simulink model "PID"  (R2023b)
settings: Solver=VariableStepAuto  StartTime=0.0  StopTime=30  RelTol=1e-3
values from neighbouring files (symbols this model uses):
  A = double(A)    [consistent.m]    (also in dyn_model_mark.m)
  B = double(B)    [consistent.m]    (also in dyn_model_mark.m)
  C = [1 0 0 0 ... (first row only)    [consistent.m]    (also in dyn_model_mark.m)
  D = [0 ... (first row only)    [consistent.m]    (also in dyn_model_mark.m)
  den_phi = cell2mat(G_t2p.Denominator)    [consistent.m]    (also in dyn_model_mark.m)
  den_theta = cell2mat(G_ol.Denominator(1,1))    [consistent.m]    (also in dyn_model_mark.m)
  Kd_phi = R_phi.Kd    [consistent.m]    (also in dyn_model_mark.m)
  Kd_theta = R_theta.Kd    [consistent.m]    (also in dyn_model_mark.m)
  Ki_phi = R_phi.Ki    [consistent.m]    (also in dyn_model_mark.m)
  Ki_theta = R_theta.Ki    [consistent.m]    (also in dyn_model_mark.m)
  Kp_phi = R_phi.Kp    [consistent.m]    (also in dyn_model_mark.m)
  Kp_theta = R_theta.Kp    [consistent.m]    (also in dyn_model_mark.m)
  num_phi = cell2mat(G_t2p.Numerator)    [consistent.m]    (also in dyn_model_mark.m)
  num_theta = cell2mat(G_ol.Numerator(1,1))    [consistent.m]    (also in dyn_model_mark.m)
  Va_bar = double(sol)    [consistent.m]    (also in dyn_model_mark.m)
  x1_bar = 0    [consistent.m]    (also in dyn_model_mark.m)
  x3_bar = 0    [consistent.m]    (also in dyn_model_mark.m = 3.14159265359)
undefined symbols (not defined in the file or in its folder): N_phi, N_theta
libraries: simulink_extras x4, slpidlib x2
settings Model: Creator=Mark  LastModifiedBy=Mark

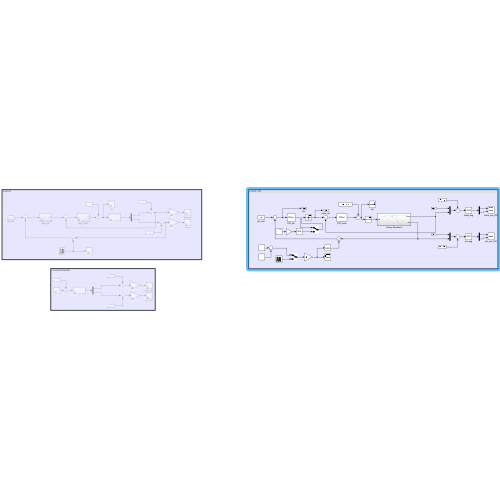
[thumbnail: Simulink's stored preview of the top-level diagram]
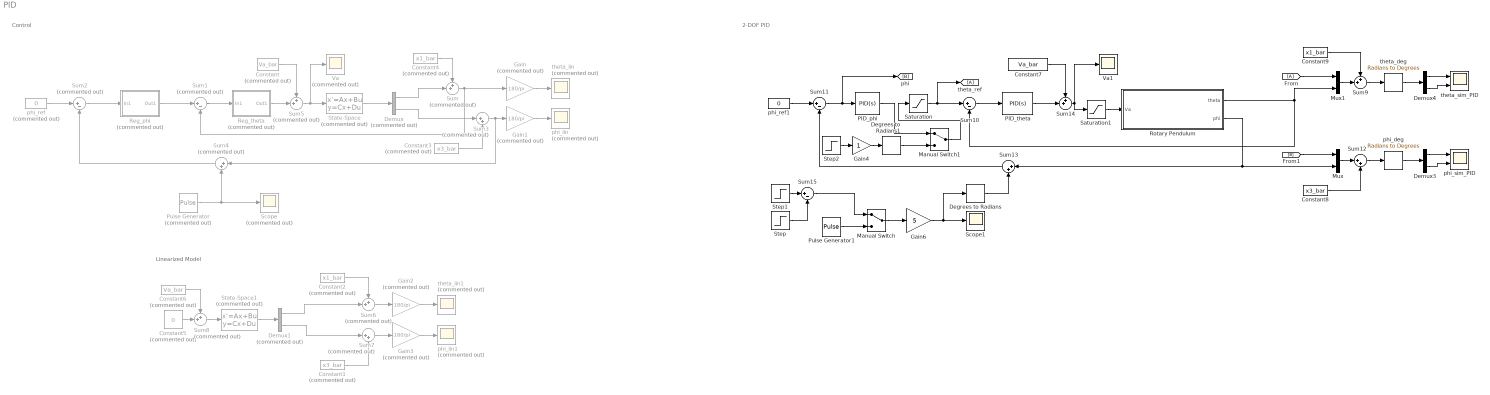
== system PID ==
  note: Control
  note: Linearized Model
  note: 2-DOF PID
  Constant : Constant  Commented=on  Value=Va_bar
  Constant1 : Constant  Commented=on  Value=x3_bar
  Constant2 : Constant  Commented=on  Value=x1_bar
  Constant3 : Constant  Commented=on  Value=x3_bar
  Constant4 : Constant  Commented=on  Value=x1_bar
  Constant5 : Constant  Commented=on  Value=0
  Constant6 : Constant  Commented=on  Value=Va_bar
  Constant7 : Constant  Value=Va_bar
  Constant8 : Constant  Value=x3_bar
  Constant9 : Constant  Value=x1_bar
  Degrees to Radians : simulink_extras/Transformations/Degrees to Radians
  Degrees to Radians1 : simulink_extras/Transformations/Degrees to Radians
  Demux : Demux  Commented=on  Outputs=2
  Demux1 : Demux  Commented=on  Outputs=2
  Demux3 : Demux  Outputs=2
  Demux4 : Demux  Outputs=2
  From : From
  Gain{,1..3} (4 alike) : Gain  Commented=on  Gain=180/pi
  Gain4 : Gain
  Gain6 : Gain  Gain=5
  Manual Switch : ManualSwitch
  Manual Switch1 : ManualSwitch
  Mux : Mux  Inputs=2
  Mux1 : Mux  Inputs=2
  PID_phi : slpidlib/PID Controller  Controller=PID  Form=Parallel  TimeDomain=Continuous-time  UseExternalTs=off  SampleTime=-1  IntegratorMethod=Forward Euler  FilterMethod=Forward Euler  ControllerParametersSource=internal  P=Kp_phi  I=Ki_phi  UseKiTs=off  D=Kd_phi  N=N_phi  UseFilter=on  TunerSelectOption=Transfer Function Based (PID Tuner App)  InitialConditionSource=internal  InitialConditionForIntegrator=0  InitialConditionForFilter=0  DifferentiatorICPrevScaledInput=0  ExternalReset=none  TrackingMode=off  Kt=1  LimitOutput=off  SatLimitsSource=internal  UpperSaturationLimit=90  LowerSaturationLimit=-90  LinearizeAsGain=on  AntiWindupMode=none  Kb=1  LimitIntegrator=off  UpperIntegratorSaturationLimit=inf  LowerIntegratorSaturationLimit=-inf  POutMin=[]  POutMax=[]  IOutMin=[]  IOutMax=[]  DOutMin=[]  DOutMax=[]  NOutMin=[]  NOutMax=[]  SumOutMin=[]  SumOutMax=[]  SaturationOutMin=[]  SaturationOutMax=[]  PParamMin=[]  PParamMax=[]  IParamMin=[]  IParamMax=[]  DParamMin=[]  DParamMax=[]  NParamMin=[]  NParamMax=[]  KbParamMin=[]  KbParamMax=[]  KtParamMin=[]  KtParamMax=[]  KbOutMin=[]  KbOutMax=[]  KtOutMin=[]  KtOutMax=[]  IntegratorOutMin=[]  IntegratorOutMax=[]  FilterOutMin=[]  FilterOutMax=[]  SumI1OutMin=[]  SumI1OutMax=[]  SumI2OutMin=[]  SumI2OutMax=[]  SumI3OutMin=[]  SumI3OutMax=[]  SumI4OutMin=[]  SumI4OutMax=[]  SumDOutMin=[]  SumDOutMax=[]  DifferentiatorOutMin=[]  DifferentiatorOutMax=[]  FilterDiffOutCoefMin=[]  FilterDiffOutCoefMax=[]  ReciprocalOutMin=[]  ReciprocalOutMax=[]  SumDenOutMin=[]  SumDenOutMax=[]  SumNumOutMin=[]  SumNumOutMax=[]  DivideOutMin=[]  DivideOutMax=[]  UdiffTsProdOutMin=[]  UdiffTsProdOutMax=[]  NTsProdOutMin=[]  NTsProdOutMax=[]  UintegralTsProdOutMin=[]  UintegralTsProdOutMax=[]  UngainTsProdOutMin=[]  UngainTsProdOutMax=[]  ClampingZeroOutDataTypeStr=Inherit: Inherit via back propagation  ClampingZeroOutMin=[]  ClampingZeroOutMax=[]  FilterDenConstantOutDataTypeStr=Inherit: Inherit via back propagation  FilterDenConstantOutMin=[]  FilterDenConstantOutMax=[]  PCopyOutDataTypeStr=Inherit: Inherit via back propagation  PCopyOutMin=[]  PCopyOutMax=[]  NCopyOutDataTypeStr=Inherit: Inherit via back propagation  NCopyOutMin=[]  NCopyOutMax=[]  IntegratorContinuousStateAttributes=''  IntegratorStateMustResolveToSignalObject=off  IntegratorRTWStateStorageClass=Auto  FilterContinuousStateAttributes=''  FilterStateMustResolveToSignalObject=off  FilterRTWStateStorageClass=Auto  ParallelPVariant=InternalParameters  IdealPVariant=Disabled  IVariant=InternalParameters  DVariant=InternalParameters  IntegratorVariant=Continuous  SatVariant=Disabled  AWVariant=Passthrough  PCopyVariant=Disabled  TRVariant=Disabled  FdbkBlocksVariant=Forward  IdealPFdbkVariant=Disabled  SatFdbkVariant=Disabled  DerivativeFilterVariant=ContFilter  NVariant=InternalParameters  NCopyVariant=Disabled  FilterICVariant=InternalICsFilter  IntegratorICVariant=InternalICs  ExternalResetVariant=Disabled  TRSumVariant=Passthrough  SumFdbkVariant=Disabled  SumVariant=Sum_PID  TsampFilterVariant=InternalTs  TsampNgainVariant=Passthrough  TsampIntegralVariant=Disabled_SignalSpec  ExternalSaturationOutDataTypeStr=Inherit: Same as second input
  PID_theta : slpidlib/PID Controller  Controller=PID  Form=Parallel  TimeDomain=Continuous-time  UseExternalTs=off  SampleTime=-1  IntegratorMethod=Forward Euler  FilterMethod=Forward Euler  ControllerParametersSource=internal  P=Kp_theta  I=Ki_theta  UseKiTs=off  D=Kd_theta  N=N_theta  UseFilter=on  TunerSelectOption=Frequency Response Based  InitialConditionSource=internal  InitialConditionForIntegrator=0  InitialConditionForFilter=0  DifferentiatorICPrevScaledInput=0  ExternalReset=none  TrackingMode=off  Kt=1  LimitOutput=off  SatLimitsSource=internal  UpperSaturationLimit=10  LowerSaturationLimit=-10  LinearizeAsGain=on  AntiWindupMode=back-calculation  Kb=Ki_theta/Kp_theta  LimitIntegrator=off  UpperIntegratorSaturationLimit=inf  LowerIntegratorSaturationLimit=-inf  POutMin=[]  POutMax=[]  IOutMin=[]  IOutMax=[]  DOutMin=[]  DOutMax=[]  NOutMin=[]  NOutMax=[]  SumOutMin=[]  SumOutMax=[]  SaturationOutMin=[]  SaturationOutMax=[]  PParamMin=[]  PParamMax=[]  IParamMin=[]  IParamMax=[]  DParamMin=[]  DParamMax=[]  NParamMin=[]  NParamMax=[]  KbParamMin=[]  KbParamMax=[]  KtParamMin=[]  KtParamMax=[]  KbOutMin=[]  KbOutMax=[]  KtOutMin=[]  KtOutMax=[]  IntegratorOutMin=[]  IntegratorOutMax=[]  FilterOutMin=[]  FilterOutMax=[]  SumI1OutMin=[]  SumI1OutMax=[]  SumI2OutMin=[]  SumI2OutMax=[]  SumI3OutMin=[]  SumI3OutMax=[]  SumI4OutMin=[]  SumI4OutMax=[]  SumDOutMin=[]  SumDOutMax=[]  DifferentiatorOutMin=[]  DifferentiatorOutMax=[]  FilterDiffOutCoefMin=[]  FilterDiffOutCoefMax=[]  ReciprocalOutMin=[]  ReciprocalOutMax=[]  SumDenOutMin=[]  SumDenOutMax=[]  SumNumOutMin=[]  SumNumOutMax=[]  DivideOutMin=[]  DivideOutMax=[]  UdiffTsProdOutMin=[]  UdiffTsProdOutMax=[]  NTsProdOutMin=[]  NTsProdOutMax=[]  UintegralTsProdOutMin=[]  UintegralTsProdOutMax=[]  UngainTsProdOutMin=[]  UngainTsProdOutMax=[]  ClampingZeroOutDataTypeStr=Inherit: Inherit via back propagation  ClampingZeroOutMin=[]  ClampingZeroOutMax=[]  FilterDenConstantOutDataTypeStr=Inherit: Inherit via back propagation  FilterDenConstantOutMin=[]  FilterDenConstantOutMax=[]  PCopyOutDataTypeStr=Inherit: Inherit via back propagation  PCopyOutMin=[]  PCopyOutMax=[]  NCopyOutDataTypeStr=Inherit: Inherit via back propagation  NCopyOutMin=[]  NCopyOutMax=[]  IntegratorContinuousStateAttributes=''  IntegratorStateMustResolveToSignalObject=off  IntegratorRTWStateStorageClass=Auto  FilterContinuousStateAttributes=''  FilterStateMustResolveToSignalObject=off  FilterRTWStateStorageClass=Auto  ParallelPVariant=InternalParameters  IdealPVariant=Disabled  IVariant=InternalParameters  DVariant=InternalParameters  IntegratorVariant=Continuous  SatVariant=Disabled  AWVariant=Passthrough  PCopyVariant=Disabled  TRVariant=Disabled  FdbkBlocksVariant=Forward  IdealPFdbkVariant=Disabled  SatFdbkVariant=Disabled  DerivativeFilterVariant=ContFilter  NVariant=InternalParameters  NCopyVariant=Disabled  FilterICVariant=InternalICsFilter  IntegratorICVariant=InternalICs  ExternalResetVariant=Disabled  TRSumVariant=Passthrough  SumFdbkVariant=Disabled  SumVariant=Sum_PID  TsampFilterVariant=InternalTs  TsampNgainVariant=Passthrough  TsampIntegralVariant=Disabled_SignalSpec  ExternalSaturationOutDataTypeStr=Inherit: Same as second input
  Pulse Generator : DiscretePulseGenerator  Commented=on  PulseType=Time based  Period=10000  PulseWidth=0.01  PhaseDelay=1
  Pulse Generator1 : DiscretePulseGenerator  PulseType=Time based  Period=10000  PulseWidth=0.005  PhaseDelay=30
  Reg_phi : Subsystem  Commented=on
  Reg_theta : Subsystem  Commented=on
  Rotary Pendulum : Subsystem
  Saturation : Saturate  UpperLimit=pi/2  LowerLimit=-pi/2
  Saturation1 : Saturate  UpperLimit=10  LowerLimit=-10
  Scope : Scope  Commented=on
  Scope1 : Scope
  State-Space : StateSpace  Commented=on  A=A  B=B  C=C  D=D  InitialCondition=[0 0 0 0]  ParameterTunability=Optimized
  State-Space1 : StateSpace  Commented=on  A=A  B=B  C=C  D=D  InitialCondition=[0 0 pi/2 0]  ParameterTunability=Optimized
  Step : Step  Time=1.05  SampleTime=0
  Step1 : Step  SampleTime=0
  Step2 : Step  SampleTime=0
  Sum{,5..6,8} (4 alike) : Sum  Commented=on  Inputs=++|
  Sum1 : Sum  Commented=on  Inputs=|+-
  Sum10 : Sum  Inputs=|+-
  Sum11 : Sum  Inputs=|+-
  Sum12 : Sum  Inputs=|++
  Sum13 : Sum  Inputs=|++
  Sum14 : Sum  Inputs=++|
  Sum15 : Sum  Inputs=|+-
  Sum2 : Sum  Commented=on  Inputs=|+-
  Sum3 : Sum  Commented=on  Inputs=|++
  Sum4 : Sum  Commented=on  Inputs=|++
  Sum7 : Sum  Commented=on  Inputs=|++
  Sum9 : Sum  Inputs=++|
  Va : Scope  Commented=on
  Va1 : Scope
  phi_deg : simulink_extras/Transformations/Radians to Degrees
  phi_lin : Scope  Commented=on
  phi_lin1 : Scope  Commented=on
  phi_ref : Constant  Commented=on  Value=0
  phi_ref1 : Constant  Value=0
  phi_sim_PID : Scope  NumInputPorts=2
  theta_deg : simulink_extras/Transformations/Radians to Degrees
  theta_lin : Scope  Commented=on
  theta_lin1 : Scope  Commented=on
  theta_ref : Goto
  theta_sim_PID : Scope  NumInputPorts=2
  wires:
  phi_ref/1 -> Sum2/1
  Reg_phi/1(Out1) -> Sum1/1
  Sum2/1 -> Reg_phi/1(In1)
  State-Space/1 -> Demux/1
  Gain/1 -> theta_lin/1
  Gain1/1 -> phi_lin/1
  Sum/1 -> Gain/1, Sum1/2
  Sum3/1 -> Sum4/1, Gain1/1
  Constant3/1 -> Sum3/2
  Constant4/1 -> Sum/1
  Demux/1 -> Sum/2
  Demux/2 -> Sum3/1
  Sum5/1 -> Va/1, State-Space/1
  Sum1/1 -> Reg_theta/1(In1)
  Sum4/1 -> Sum2/2
  Pulse Generator/1 -> Scope/1, Sum4/2
  Reg_theta/1(Out1) -> Sum5/2
  Constant/1 -> Sum5/1
  Demux1/2 -> Sum7/1
  Sum7/1 -> Gain3/1
  Gain3/1 -> phi_lin1/1
  State-Space1/1 -> Demux1/1
  Demux1/1 -> Sum6/2
  Constant2/1 -> Sum6/1
  Gain2/1 -> theta_lin1/1
  Constant1/1 -> Sum7/2
  Sum6/1 -> Gain2/1
  Constant5/1 -> Sum8/2
  Sum8/1 -> State-Space1/1
  Constant6/1 -> Sum8/1
  phi_ref1/1 -> Sum11/1
  Sum13/1 -> Sum11/2
  Sum10/1 -> PID_theta/1
  Constant9/1 -> Sum9/1
  Manual Switch/1 -> Gain6/1
  Sum11/1 -> [B], PID_phi/1
  Constant8/1 -> Sum12/2
  Constant7/1 -> Sum14/1
  Gain6/1 -> Scope1/1, Degrees to Radians/1
  From/1 -> Mux1/1
  [B] -> Mux/1
  Pulse Generator1/1 -> Manual Switch/2
  PID_theta/1 -> Sum14/2
  Sum12/1 -> phi_deg/1
  Sum14/1 -> Saturation1/1, Va1/1
  Manual Switch1/1 -> Saturation/1
  phi_deg/1 -> Demux3/1
  Degrees to Radians/1 -> Sum13/2
  Mux/1 -> Sum12/1
  Demux3/1 -> phi_sim_PID/1
  Demux3/2 -> phi_sim_PID/2
  Mux1/1 -> Sum9/2
  theta_deg/1 -> Demux4/1
  Demux4/1 -> theta_sim_PID/1
  Demux4/2 -> theta_sim_PID/2
  Sum9/1 -> theta_deg/1
  Rotary Pendulum/1(theta) -> Mux1/2, Sum10/2
  Rotary Pendulum/2(phi) -> Sum13/1, Mux/2
  Sum15/1 -> Manual Switch/1
  Step/1 -> Sum15/2
  Step1/1 -> Sum15/1
  Saturation/1 -> theta_ref/1, Sum10/1
  Saturation1/1 -> Rotary Pendulum/1(Va)
  Step2/1 -> Gain4/1
  PID_phi/1 -> Manual Switch1/1
  Degrees to Radians1/1 -> Manual Switch1/2
  Gain4/1 -> Degrees to Radians1/1

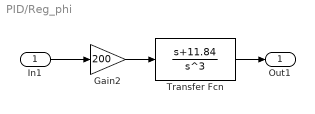
== system PID/Reg_phi ==
  In1 : Inport
  Gain2 : Gain  Gain=200
  Transfer Fcn : TransferFcn  Numerator=[1 11.84]  Denominator=[1 0 0 0]
  Out1 : Outport
  wires:
  Gain2/1 -> Transfer Fcn/1
  Transfer Fcn/1 -> Out1/1
  In1/1 -> Gain2/1

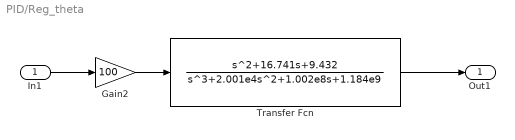
== system PID/Reg_theta ==
  In1 : Inport
  Gain2 : Gain  Gain=100
  Transfer Fcn : TransferFcn  Numerator=[1 16.741 9.432]  Denominator=[1 2.001e4 1.002e8 1.184e9]
  Out1 : Outport
  wires:
  Gain2/1 -> Transfer Fcn/1
  Transfer Fcn/1 -> Out1/1
  In1/1 -> Gain2/1

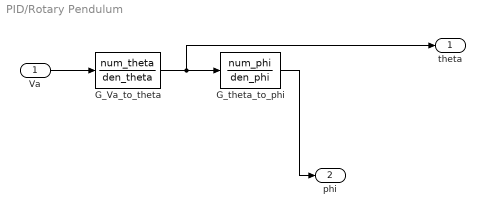
== system PID/Rotary Pendulum ==
  Va : Inport
  G_Va_to_theta : TransferFcn  Numerator=num_theta  Denominator=den_theta
  G_theta_to_phi : TransferFcn  Numerator=num_phi  Denominator=den_phi
  theta : Outport
  phi : Outport  Port=2
  wires:
  G_theta_to_phi/1 -> phi/1
  G_Va_to_theta/1 -> theta/1, G_theta_to_phi/1
  Va/1 -> G_Va_to_theta/1
